simulink model "tracker"  (R2020a)
settings: Solver=VariableStepAuto  StartTime=0.0  StopTime=simulation_time  RelTol=1e-3
values from neighbouring files (symbols this model uses):
  costas_pll_arctan_nstage = 8    [tracker_hw_init.m]
  costas_pll_arctan_point = 16    [tracker_hw_init.m]
  costas_pll_arctan_width = 32    [tracker_hw_init.m]
  DDS_ch_pinc = fc.*(2^(DDS_phase_width)/fs)    [tracker_hw_init.m]
  fs = 120e6    (= 120000000)    [tracker_hw_init.m]
  normalized_EML_power_cordic_nstage = 11    [tracker_hw_init.m]
  normalized_EML_power_cordic_point = 32    [tracker_hw_init.m]
  normalized_EML_power_cordic_width = 32    [tracker_hw_init.m]
  ts = 1/fs    (= 8.33333333333e-09)    [tracker_hw_init.m]
undefined symbols (not defined in the file or in its folder): cacode, i
libraries: xbsIndex_r4 x1873
(part 4 of 14)

== system tracker/CA_code_bank/input_router/address_router32 ==
  ca_select : Inport
  Mux{,1..10} (11 alike) : xbsIndex_r4/Mux  inputs=2  en=off  latency=1  precision=Full  arith_type=Unsigned  n_bits=16  bin_pt=14  quantization=Truncate  overflow=Wrap  dbl_ovrd=off  block_type=mux
  Relational{,1..10} (11 alike) : xbsIndex_r4/Relational  mode=a=b  op_type=Bool  en=off  latency=1  dbl_ovrd=off  block_type=relational
  ca_addr : Outport
  wires:
  [CA_code_addr_ch11] -> Mux10/3
  Mux8/1 -> Mux7/2
  Mux5/1 -> Mux4/2
  [CA_code_select_ch8] -> Relational7/1
  [CA_code_addr_ch9] -> Mux8/3
  [CA_code_select_ch7] -> Relational6/1
  Relational/1 -> Mux/1
  [CA_code_addr_ch1] -> Mux/3
  Mux9/1 -> Mux8/2
  ca_select/1 -> Relational1/2, Relational2/2, Relational3/2, Relational4/2, Relational5/2, Relational6/2, Relational7/2, Relational8/2, Relational9/2, Relational10/2, Relational/2
  Relational9/1 -> Mux9/1
  Mux3/1 -> Mux2/2
  [CA_code_select_ch4] -> Relational3/1
  [CA_code_select_ch3] -> Relational2/1
  Relational8/1 -> Mux8/1
  Relational2/1 -> Mux2/1
  [CA_code_addr_ch5] -> Mux4/3
  [CA_code_select_ch5] -> Relational4/1
  Relational10/1 -> Mux10/1
  Mux2/1 -> Mux1/2
  [CA_code_select_ch2] -> Relational1/1
  Mux4/1 -> Mux3/2
  Relational7/1 -> Mux7/1
  Relational4/1 -> Mux4/1
  [CA_code_select_ch6] -> Relational5/1
  [CA_code_addr_ch6] -> Mux5/3
  [CA_code_addr_ch3] -> Mux2/3
  [CA_code_select_ch1] -> Relational/1
  [CA_code_addr_ch4] -> Mux3/3
  Relational3/1 -> Mux3/1
  [CA_code_select_ch11] -> Relational10/1
  [CA_code_select_ch10] -> Relational9/1
  [CA_code_select_ch9] -> Relational8/1
  Relational5/1 -> Mux5/1
  Mux10/1 -> Mux9/2
  [CA_code_addr_ch10] -> Mux9/3
  Mux7/1 -> Mux6/2
  [CA_code_addr_ch12] -> Mux10/2
  Relational1/1 -> Mux1/1
  [CA_code_addr_ch8] -> Mux7/3
  [CA_code_addr_ch7] -> Mux6/3
  Mux1/1 -> Mux/2
  [CA_code_addr_ch2] -> Mux1/3
  Relational6/1 -> Mux6/1
  Mux6/1 -> Mux5/2
  Mux/1 -> ca_addr/1

== system tracker/CA_code_bank/input_router/address_router33 ==
  ca_select : Inport
  Mux{,1..10} (11 alike) : xbsIndex_r4/Mux  inputs=2  en=off  latency=1  precision=Full  arith_type=Unsigned  n_bits=16  bin_pt=14  quantization=Truncate  overflow=Wrap  dbl_ovrd=off  block_type=mux
  Relational{,1..10} (11 alike) : xbsIndex_r4/Relational  mode=a=b  op_type=Bool  en=off  latency=1  dbl_ovrd=off  block_type=relational
  ca_addr : Outport
  wires:
  Mux/1 -> ca_addr/1
  Mux6/1 -> Mux5/2
  Relational6/1 -> Mux6/1
  [CA_code_addr_ch2] -> Mux1/3
  Mux1/1 -> Mux/2
  [CA_code_addr_ch7] -> Mux6/3
  [CA_code_addr_ch8] -> Mux7/3
  Relational1/1 -> Mux1/1
  [CA_code_addr_ch12] -> Mux10/2
  Mux7/1 -> Mux6/2
  [CA_code_addr_ch10] -> Mux9/3
  Mux10/1 -> Mux9/2
  Relational5/1 -> Mux5/1
  [CA_code_select_ch9] -> Relational8/1
  [CA_code_select_ch10] -> Relational9/1
  [CA_code_select_ch11] -> Relational10/1
  Relational3/1 -> Mux3/1
  [CA_code_addr_ch4] -> Mux3/3
  [CA_code_select_ch1] -> Relational/1
  [CA_code_addr_ch3] -> Mux2/3
  [CA_code_addr_ch6] -> Mux5/3
  [CA_code_select_ch6] -> Relational5/1
  Relational4/1 -> Mux4/1
  Relational7/1 -> Mux7/1
  Mux4/1 -> Mux3/2
  [CA_code_select_ch2] -> Relational1/1
  Mux2/1 -> Mux1/2
  Relational10/1 -> Mux10/1
  [CA_code_select_ch5] -> Relational4/1
  [CA_code_addr_ch5] -> Mux4/3
  Relational2/1 -> Mux2/1
  Relational8/1 -> Mux8/1
  [CA_code_select_ch3] -> Relational2/1
  [CA_code_select_ch4] -> Relational3/1
  Mux3/1 -> Mux2/2
  Relational9/1 -> Mux9/1
  ca_select/1 -> Relational/2, Relational10/2, Relational9/2, Relational8/2, Relational7/2, Relational6/2, Relational5/2, Relational4/2, Relational3/2, Relational2/2, Relational1/2
  Mux9/1 -> Mux8/2
  [CA_code_addr_ch1] -> Mux/3
  Relational/1 -> Mux/1
  [CA_code_select_ch7] -> Relational6/1
  [CA_code_addr_ch9] -> Mux8/3
  [CA_code_select_ch8] -> Relational7/1
  Mux5/1 -> Mux4/2
  Mux8/1 -> Mux7/2
  [CA_code_addr_ch11] -> Mux10/3

== system tracker/CA_code_bank/input_router/address_router34 ==
  ca_select : Inport
  Mux{,1..10} (11 alike) : xbsIndex_r4/Mux  inputs=2  en=off  latency=1  precision=Full  arith_type=Unsigned  n_bits=16  bin_pt=14  quantization=Truncate  overflow=Wrap  dbl_ovrd=off  block_type=mux
  Relational{,1..10} (11 alike) : xbsIndex_r4/Relational  mode=a=b  op_type=Bool  en=off  latency=1  dbl_ovrd=off  block_type=relational
  ca_addr : Outport
  wires:
  Mux/1 -> ca_addr/1
  Mux6/1 -> Mux5/2
  Relational6/1 -> Mux6/1
  [CA_code_addr_ch2] -> Mux1/3
  Mux1/1 -> Mux/2
  [CA_code_addr_ch7] -> Mux6/3
  [CA_code_addr_ch8] -> Mux7/3
  Relational1/1 -> Mux1/1
  [CA_code_addr_ch12] -> Mux10/2
  Mux7/1 -> Mux6/2
  [CA_code_addr_ch10] -> Mux9/3
  Mux10/1 -> Mux9/2
  Relational5/1 -> Mux5/1
  [CA_code_select_ch9] -> Relational8/1
  [CA_code_select_ch10] -> Relational9/1
  [CA_code_select_ch11] -> Relational10/1
  Relational3/1 -> Mux3/1
  [CA_code_addr_ch4] -> Mux3/3
  [CA_code_select_ch1] -> Relational/1
  [CA_code_addr_ch3] -> Mux2/3
  [CA_code_addr_ch6] -> Mux5/3
  [CA_code_select_ch6] -> Relational5/1
  Relational4/1 -> Mux4/1
  Relational7/1 -> Mux7/1
  Mux4/1 -> Mux3/2
  [CA_code_select_ch2] -> Relational1/1
  Mux2/1 -> Mux1/2
  Relational10/1 -> Mux10/1
  [CA_code_select_ch5] -> Relational4/1
  [CA_code_addr_ch5] -> Mux4/3
  Relational2/1 -> Mux2/1
  Relational8/1 -> Mux8/1
  [CA_code_select_ch3] -> Relational2/1
  [CA_code_select_ch4] -> Relational3/1
  Mux3/1 -> Mux2/2
  Relational9/1 -> Mux9/1
  ca_select/1 -> Relational/2, Relational10/2, Relational9/2, Relational8/2, Relational7/2, Relational6/2, Relational5/2, Relational4/2, Relational3/2, Relational2/2, Relational1/2
  Mux9/1 -> Mux8/2
  [CA_code_addr_ch1] -> Mux/3
  Relational/1 -> Mux/1
  [CA_code_select_ch7] -> Relational6/1
  [CA_code_addr_ch9] -> Mux8/3
  [CA_code_select_ch8] -> Relational7/1
  Mux5/1 -> Mux4/2
  Mux8/1 -> Mux7/2
  [CA_code_addr_ch11] -> Mux10/3

== system tracker/CA_code_bank/input_router/address_router35 ==
  ca_select : Inport
  Mux{,1..10} (11 alike) : xbsIndex_r4/Mux  inputs=2  en=off  latency=1  precision=Full  arith_type=Unsigned  n_bits=16  bin_pt=14  quantization=Truncate  overflow=Wrap  dbl_ovrd=off  block_type=mux
  Relational{,1..10} (11 alike) : xbsIndex_r4/Relational  mode=a=b  op_type=Bool  en=off  latency=1  dbl_ovrd=off  block_type=relational
  ca_addr : Outport
  wires:
  [CA_code_addr_ch11] -> Mux10/3
  Mux8/1 -> Mux7/2
  Mux5/1 -> Mux4/2
  [CA_code_select_ch8] -> Relational7/1
  [CA_code_addr_ch9] -> Mux8/3
  [CA_code_select_ch7] -> Relational6/1
  Relational/1 -> Mux/1
  [CA_code_addr_ch1] -> Mux/3
  Mux9/1 -> Mux8/2
  ca_select/1 -> Relational1/2, Relational2/2, Relational3/2, Relational4/2, Relational5/2, Relational6/2, Relational7/2, Relational8/2, Relational9/2, Relational10/2, Relational/2
  Relational9/1 -> Mux9/1
  Mux3/1 -> Mux2/2
  [CA_code_select_ch4] -> Relational3/1
  [CA_code_select_ch3] -> Relational2/1
  Relational8/1 -> Mux8/1
  Relational2/1 -> Mux2/1
  [CA_code_addr_ch5] -> Mux4/3
  [CA_code_select_ch5] -> Relational4/1
  Relational10/1 -> Mux10/1
  Mux2/1 -> Mux1/2
  [CA_code_select_ch2] -> Relational1/1
  Mux4/1 -> Mux3/2
  Relational7/1 -> Mux7/1
  Relational4/1 -> Mux4/1
  [CA_code_select_ch6] -> Relational5/1
  [CA_code_addr_ch6] -> Mux5/3
  [CA_code_addr_ch3] -> Mux2/3
  [CA_code_select_ch1] -> Relational/1
  [CA_code_addr_ch4] -> Mux3/3
  Relational3/1 -> Mux3/1
  [CA_code_select_ch11] -> Relational10/1
  [CA_code_select_ch10] -> Relational9/1
  [CA_code_select_ch9] -> Relational8/1
  Relational5/1 -> Mux5/1
  Mux10/1 -> Mux9/2
  [CA_code_addr_ch10] -> Mux9/3
  Mux7/1 -> Mux6/2
  [CA_code_addr_ch12] -> Mux10/2
  Relational1/1 -> Mux1/1
  [CA_code_addr_ch8] -> Mux7/3
  [CA_code_addr_ch7] -> Mux6/3
  Mux1/1 -> Mux/2
  [CA_code_addr_ch2] -> Mux1/3
  Relational6/1 -> Mux6/1
  Mux6/1 -> Mux5/2
  Mux/1 -> ca_addr/1

== system tracker/CA_code_bank/input_router/address_router36 ==
  ca_select : Inport
  Mux{,1..10} (11 alike) : xbsIndex_r4/Mux  inputs=2  en=off  latency=1  precision=Full  arith_type=Unsigned  n_bits=16  bin_pt=14  quantization=Truncate  overflow=Wrap  dbl_ovrd=off  block_type=mux
  Relational{,1..10} (11 alike) : xbsIndex_r4/Relational  mode=a=b  op_type=Bool  en=off  latency=1  dbl_ovrd=off  block_type=relational
  ca_addr : Outport
  wires:
  Mux/1 -> ca_addr/1
  Mux6/1 -> Mux5/2
  Relational6/1 -> Mux6/1
  [CA_code_addr_ch2] -> Mux1/3
  Mux1/1 -> Mux/2
  [CA_code_addr_ch7] -> Mux6/3
  [CA_code_addr_ch8] -> Mux7/3
  Relational1/1 -> Mux1/1
  [CA_code_addr_ch12] -> Mux10/2
  Mux7/1 -> Mux6/2
  [CA_code_addr_ch10] -> Mux9/3
  Mux10/1 -> Mux9/2
  Relational5/1 -> Mux5/1
  [CA_code_select_ch9] -> Relational8/1
  [CA_code_select_ch10] -> Relational9/1
  [CA_code_select_ch11] -> Relational10/1
  Relational3/1 -> Mux3/1
  [CA_code_addr_ch4] -> Mux3/3
  [CA_code_select_ch1] -> Relational/1
  [CA_code_addr_ch3] -> Mux2/3
  [CA_code_addr_ch6] -> Mux5/3
  [CA_code_select_ch6] -> Relational5/1
  Relational4/1 -> Mux4/1
  Relational7/1 -> Mux7/1
  Mux4/1 -> Mux3/2
  [CA_code_select_ch2] -> Relational1/1
  Mux2/1 -> Mux1/2
  Relational10/1 -> Mux10/1
  [CA_code_select_ch5] -> Relational4/1
  [CA_code_addr_ch5] -> Mux4/3
  Relational2/1 -> Mux2/1
  Relational8/1 -> Mux8/1
  [CA_code_select_ch3] -> Relational2/1
  [CA_code_select_ch4] -> Relational3/1
  Mux3/1 -> Mux2/2
  Relational9/1 -> Mux9/1
  ca_select/1 -> Relational/2, Relational10/2, Relational9/2, Relational8/2, Relational7/2, Relational6/2, Relational5/2, Relational4/2, Relational3/2, Relational2/2, Relational1/2
  Mux9/1 -> Mux8/2
  [CA_code_addr_ch1] -> Mux/3
  Relational/1 -> Mux/1
  [CA_code_select_ch7] -> Relational6/1
  [CA_code_addr_ch9] -> Mux8/3
  [CA_code_select_ch8] -> Relational7/1
  Mux5/1 -> Mux4/2
  Mux8/1 -> Mux7/2
  [CA_code_addr_ch11] -> Mux10/3

== system tracker/CA_code_bank/input_router/address_router37 ==
  ca_select : Inport
  Mux{,1..10} (11 alike) : xbsIndex_r4/Mux  inputs=2  en=off  latency=1  precision=Full  arith_type=Unsigned  n_bits=16  bin_pt=14  quantization=Truncate  overflow=Wrap  dbl_ovrd=off  block_type=mux
  Relational{,1..10} (11 alike) : xbsIndex_r4/Relational  mode=a=b  op_type=Bool  en=off  latency=1  dbl_ovrd=off  block_type=relational
  ca_addr : Outport
  wires:
  Mux/1 -> ca_addr/1
  Mux6/1 -> Mux5/2
  Relational6/1 -> Mux6/1
  [CA_code_addr_ch2] -> Mux1/3
  Mux1/1 -> Mux/2
  [CA_code_addr_ch7] -> Mux6/3
  [CA_code_addr_ch8] -> Mux7/3
  Relational1/1 -> Mux1/1
  [CA_code_addr_ch12] -> Mux10/2
  Mux7/1 -> Mux6/2
  [CA_code_addr_ch10] -> Mux9/3
  Mux10/1 -> Mux9/2
  Relational5/1 -> Mux5/1
  [CA_code_select_ch9] -> Relational8/1
  [CA_code_select_ch10] -> Relational9/1
  [CA_code_select_ch11] -> Relational10/1
  Relational3/1 -> Mux3/1
  [CA_code_addr_ch4] -> Mux3/3
  [CA_code_select_ch1] -> Relational/1
  [CA_code_addr_ch3] -> Mux2/3
  [CA_code_addr_ch6] -> Mux5/3
  [CA_code_select_ch6] -> Relational5/1
  Relational4/1 -> Mux4/1
  Relational7/1 -> Mux7/1
  Mux4/1 -> Mux3/2
  [CA_code_select_ch2] -> Relational1/1
  Mux2/1 -> Mux1/2
  Relational10/1 -> Mux10/1
  [CA_code_select_ch5] -> Relational4/1
  [CA_code_addr_ch5] -> Mux4/3
  Relational2/1 -> Mux2/1
  Relational8/1 -> Mux8/1
  [CA_code_select_ch3] -> Relational2/1
  [CA_code_select_ch4] -> Relational3/1
  Mux3/1 -> Mux2/2
  Relational9/1 -> Mux9/1
  ca_select/1 -> Relational/2, Relational10/2, Relational9/2, Relational8/2, Relational7/2, Relational6/2, Relational5/2, Relational4/2, Relational3/2, Relational2/2, Relational1/2
  Mux9/1 -> Mux8/2
  [CA_code_addr_ch1] -> Mux/3
  Relational/1 -> Mux/1
  [CA_code_select_ch7] -> Relational6/1
  [CA_code_addr_ch9] -> Mux8/3
  [CA_code_select_ch8] -> Relational7/1
  Mux5/1 -> Mux4/2
  Mux8/1 -> Mux7/2
  [CA_code_addr_ch11] -> Mux10/3

== system tracker/CA_code_bank/input_router/address_router4 ==
  ca_select : Inport
  Mux{,1..10} (11 alike) : xbsIndex_r4/Mux  inputs=2  en=off  latency=1  precision=Full  arith_type=Unsigned  n_bits=16  bin_pt=14  quantization=Truncate  overflow=Wrap  dbl_ovrd=off  block_type=mux
  Relational{,1..10} (11 alike) : xbsIndex_r4/Relational  mode=a=b  op_type=Bool  en=off  latency=1  dbl_ovrd=off  block_type=relational
  ca_addr : Outport
  wires:
  Mux/1 -> ca_addr/1
  Mux6/1 -> Mux5/2
  Relational6/1 -> Mux6/1
  [CA_code_addr_ch2] -> Mux1/3
  Mux1/1 -> Mux/2
  [CA_code_addr_ch7] -> Mux6/3
  [CA_code_addr_ch8] -> Mux7/3
  Relational1/1 -> Mux1/1
  [CA_code_addr_ch12] -> Mux10/2
  Mux7/1 -> Mux6/2
  [CA_code_addr_ch10] -> Mux9/3
  Mux10/1 -> Mux9/2
  Relational5/1 -> Mux5/1
  [CA_code_select_ch9] -> Relational8/1
  [CA_code_select_ch10] -> Relational9/1
  [CA_code_select_ch11] -> Relational10/1
  Relational3/1 -> Mux3/1
  [CA_code_addr_ch4] -> Mux3/3
  [CA_code_select_ch1] -> Relational/1
  [CA_code_addr_ch3] -> Mux2/3
  [CA_code_addr_ch6] -> Mux5/3
  [CA_code_select_ch6] -> Relational5/1
  Relational4/1 -> Mux4/1
  Relational7/1 -> Mux7/1
  Mux4/1 -> Mux3/2
  [CA_code_select_ch2] -> Relational1/1
  Mux2/1 -> Mux1/2
  Relational10/1 -> Mux10/1
  [CA_code_select_ch5] -> Relational4/1
  [CA_code_addr_ch5] -> Mux4/3
  Relational2/1 -> Mux2/1
  Relational8/1 -> Mux8/1
  [CA_code_select_ch3] -> Relational2/1
  [CA_code_select_ch4] -> Relational3/1
  Mux3/1 -> Mux2/2
  Relational9/1 -> Mux9/1
  ca_select/1 -> Relational/2, Relational10/2, Relational9/2, Relational8/2, Relational7/2, Relational6/2, Relational5/2, Relational4/2, Relational3/2, Relational2/2, Relational1/2
  Mux9/1 -> Mux8/2
  [CA_code_addr_ch1] -> Mux/3
  Relational/1 -> Mux/1
  [CA_code_select_ch7] -> Relational6/1
  [CA_code_addr_ch9] -> Mux8/3
  [CA_code_select_ch8] -> Relational7/1
  Mux5/1 -> Mux4/2
  Mux8/1 -> Mux7/2
  [CA_code_addr_ch11] -> Mux10/3

== system tracker/CA_code_bank/input_router/address_router5 ==
  ca_select : Inport
  Mux{,1..10} (11 alike) : xbsIndex_r4/Mux  inputs=2  en=off  latency=1  precision=Full  arith_type=Unsigned  n_bits=16  bin_pt=14  quantization=Truncate  overflow=Wrap  dbl_ovrd=off  block_type=mux
  Relational{,1..10} (11 alike) : xbsIndex_r4/Relational  mode=a=b  op_type=Bool  en=off  latency=1  dbl_ovrd=off  block_type=relational
  ca_addr : Outport
  wires:
  [CA_code_addr_ch11] -> Mux10/3
  Mux8/1 -> Mux7/2
  Mux5/1 -> Mux4/2
  [CA_code_select_ch8] -> Relational7/1
  [CA_code_addr_ch9] -> Mux8/3
  [CA_code_select_ch7] -> Relational6/1
  Relational/1 -> Mux/1
  [CA_code_addr_ch1] -> Mux/3
  Mux9/1 -> Mux8/2
  ca_select/1 -> Relational1/2, Relational2/2, Relational3/2, Relational4/2, Relational5/2, Relational6/2, Relational7/2, Relational8/2, Relational9/2, Relational10/2, Relational/2
  Relational9/1 -> Mux9/1
  Mux3/1 -> Mux2/2
  [CA_code_select_ch4] -> Relational3/1
  [CA_code_select_ch3] -> Relational2/1
  Relational8/1 -> Mux8/1
  Relational2/1 -> Mux2/1
  [CA_code_addr_ch5] -> Mux4/3
  [CA_code_select_ch5] -> Relational4/1
  Relational10/1 -> Mux10/1
  Mux2/1 -> Mux1/2
  [CA_code_select_ch2] -> Relational1/1
  Mux4/1 -> Mux3/2
  Relational7/1 -> Mux7/1
  Relational4/1 -> Mux4/1
  [CA_code_select_ch6] -> Relational5/1
  [CA_code_addr_ch6] -> Mux5/3
  [CA_code_addr_ch3] -> Mux2/3
  [CA_code_select_ch1] -> Relational/1
  [CA_code_addr_ch4] -> Mux3/3
  Relational3/1 -> Mux3/1
  [CA_code_select_ch11] -> Relational10/1
  [CA_code_select_ch10] -> Relational9/1
  [CA_code_select_ch9] -> Relational8/1
  Relational5/1 -> Mux5/1
  Mux10/1 -> Mux9/2
  [CA_code_addr_ch10] -> Mux9/3
  Mux7/1 -> Mux6/2
  [CA_code_addr_ch12] -> Mux10/2
  Relational1/1 -> Mux1/1
  [CA_code_addr_ch8] -> Mux7/3
  [CA_code_addr_ch7] -> Mux6/3
  Mux1/1 -> Mux/2
  [CA_code_addr_ch2] -> Mux1/3
  Relational6/1 -> Mux6/1
  Mux6/1 -> Mux5/2
  Mux/1 -> ca_addr/1

== system tracker/CA_code_bank/input_router/address_router6 ==
  ca_select : Inport
  Mux{,1..10} (11 alike) : xbsIndex_r4/Mux  inputs=2  en=off  latency=1  precision=Full  arith_type=Unsigned  n_bits=16  bin_pt=14  quantization=Truncate  overflow=Wrap  dbl_ovrd=off  block_type=mux
  Relational{,1..10} (11 alike) : xbsIndex_r4/Relational  mode=a=b  op_type=Bool  en=off  latency=1  dbl_ovrd=off  block_type=relational
  ca_addr : Outport
  wires:
  Mux/1 -> ca_addr/1
  Mux6/1 -> Mux5/2
  Relational6/1 -> Mux6/1
  [CA_code_addr_ch2] -> Mux1/3
  Mux1/1 -> Mux/2
  [CA_code_addr_ch7] -> Mux6/3
  [CA_code_addr_ch8] -> Mux7/3
  Relational1/1 -> Mux1/1
  [CA_code_addr_ch12] -> Mux10/2
  Mux7/1 -> Mux6/2
  [CA_code_addr_ch10] -> Mux9/3
  Mux10/1 -> Mux9/2
  Relational5/1 -> Mux5/1
  [CA_code_select_ch9] -> Relational8/1
  [CA_code_select_ch10] -> Relational9/1
  [CA_code_select_ch11] -> Relational10/1
  Relational3/1 -> Mux3/1
  [CA_code_addr_ch4] -> Mux3/3
  [CA_code_select_ch1] -> Relational/1
  [CA_code_addr_ch3] -> Mux2/3
  [CA_code_addr_ch6] -> Mux5/3
  [CA_code_select_ch6] -> Relational5/1
  Relational4/1 -> Mux4/1
  Relational7/1 -> Mux7/1
  Mux4/1 -> Mux3/2
  [CA_code_select_ch2] -> Relational1/1
  Mux2/1 -> Mux1/2
  Relational10/1 -> Mux10/1
  [CA_code_select_ch5] -> Relational4/1
  [CA_code_addr_ch5] -> Mux4/3
  Relational2/1 -> Mux2/1
  Relational8/1 -> Mux8/1
  [CA_code_select_ch3] -> Relational2/1
  [CA_code_select_ch4] -> Relational3/1
  Mux3/1 -> Mux2/2
  Relational9/1 -> Mux9/1
  ca_select/1 -> Relational/2, Relational10/2, Relational9/2, Relational8/2, Relational7/2, Relational6/2, Relational5/2, Relational4/2, Relational3/2, Relational2/2, Relational1/2
  Mux9/1 -> Mux8/2
  [CA_code_addr_ch1] -> Mux/3
  Relational/1 -> Mux/1
  [CA_code_select_ch7] -> Relational6/1
  [CA_code_addr_ch9] -> Mux8/3
  [CA_code_select_ch8] -> Relational7/1
  Mux5/1 -> Mux4/2
  Mux8/1 -> Mux7/2
  [CA_code_addr_ch11] -> Mux10/3

== system tracker/CA_code_bank/input_router/address_router7 ==
  ca_select : Inport
  Mux{,1..10} (11 alike) : xbsIndex_r4/Mux  inputs=2  en=off  latency=1  precision=Full  arith_type=Unsigned  n_bits=16  bin_pt=14  quantization=Truncate  overflow=Wrap  dbl_ovrd=off  block_type=mux
  Relational{,1..10} (11 alike) : xbsIndex_r4/Relational  mode=a=b  op_type=Bool  en=off  latency=1  dbl_ovrd=off  block_type=relational
  ca_addr : Outport
  wires:
  Mux/1 -> ca_addr/1
  Mux6/1 -> Mux5/2
  Relational6/1 -> Mux6/1
  [CA_code_addr_ch2] -> Mux1/3
  Mux1/1 -> Mux/2
  [CA_code_addr_ch7] -> Mux6/3
  [CA_code_addr_ch8] -> Mux7/3
  Relational1/1 -> Mux1/1
  [CA_code_addr_ch12] -> Mux10/2
  Mux7/1 -> Mux6/2
  [CA_code_addr_ch10] -> Mux9/3
  Mux10/1 -> Mux9/2
  Relational5/1 -> Mux5/1
  [CA_code_select_ch9] -> Relational8/1
  [CA_code_select_ch10] -> Relational9/1
  [CA_code_select_ch11] -> Relational10/1
  Relational3/1 -> Mux3/1
  [CA_code_addr_ch4] -> Mux3/3
  [CA_code_select_ch1] -> Relational/1
  [CA_code_addr_ch3] -> Mux2/3
  [CA_code_addr_ch6] -> Mux5/3
  [CA_code_select_ch6] -> Relational5/1
  Relational4/1 -> Mux4/1
  Relational7/1 -> Mux7/1
  Mux4/1 -> Mux3/2
  [CA_code_select_ch2] -> Relational1/1
  Mux2/1 -> Mux1/2
  Relational10/1 -> Mux10/1
  [CA_code_select_ch5] -> Relational4/1
  [CA_code_addr_ch5] -> Mux4/3
  Relational2/1 -> Mux2/1
  Relational8/1 -> Mux8/1
  [CA_code_select_ch3] -> Relational2/1
  [CA_code_select_ch4] -> Relational3/1
  Mux3/1 -> Mux2/2
  Relational9/1 -> Mux9/1
  ca_select/1 -> Relational/2, Relational10/2, Relational9/2, Relational8/2, Relational7/2, Relational6/2, Relational5/2, Relational4/2, Relational3/2, Relational2/2, Relational1/2
  Mux9/1 -> Mux8/2
  [CA_code_addr_ch1] -> Mux/3
  Relational/1 -> Mux/1
  [CA_code_select_ch7] -> Relational6/1
  [CA_code_addr_ch9] -> Mux8/3
  [CA_code_select_ch8] -> Relational7/1
  Mux5/1 -> Mux4/2
  Mux8/1 -> Mux7/2
  [CA_code_addr_ch11] -> Mux10/3

== system tracker/CA_code_bank/input_router/address_router8 ==
  ca_select : Inport
  Mux{,1..10} (11 alike) : xbsIndex_r4/Mux  inputs=2  en=off  latency=1  precision=Full  arith_type=Unsigned  n_bits=16  bin_pt=14  quantization=Truncate  overflow=Wrap  dbl_ovrd=off  block_type=mux
  Relational{,1..10} (11 alike) : xbsIndex_r4/Relational  mode=a=b  op_type=Bool  en=off  latency=1  dbl_ovrd=off  block_type=relational
  ca_addr : Outport
  wires:
  [CA_code_addr_ch11] -> Mux10/3
  Mux8/1 -> Mux7/2
  Mux5/1 -> Mux4/2
  [CA_code_select_ch8] -> Relational7/1
  [CA_code_addr_ch9] -> Mux8/3
  [CA_code_select_ch7] -> Relational6/1
  Relational/1 -> Mux/1
  [CA_code_addr_ch1] -> Mux/3
  Mux9/1 -> Mux8/2
  ca_select/1 -> Relational1/2, Relational2/2, Relational3/2, Relational4/2, Relational5/2, Relational6/2, Relational7/2, Relational8/2, Relational9/2, Relational10/2, Relational/2
  Relational9/1 -> Mux9/1
  Mux3/1 -> Mux2/2
  [CA_code_select_ch4] -> Relational3/1
  [CA_code_select_ch3] -> Relational2/1
  Relational8/1 -> Mux8/1
  Relational2/1 -> Mux2/1
  [CA_code_addr_ch5] -> Mux4/3
  [CA_code_select_ch5] -> Relational4/1
  Relational10/1 -> Mux10/1
  Mux2/1 -> Mux1/2
  [CA_code_select_ch2] -> Relational1/1
  Mux4/1 -> Mux3/2
  Relational7/1 -> Mux7/1
  Relational4/1 -> Mux4/1
  [CA_code_select_ch6] -> Relational5/1
  [CA_code_addr_ch6] -> Mux5/3
  [CA_code_addr_ch3] -> Mux2/3
  [CA_code_select_ch1] -> Relational/1
  [CA_code_addr_ch4] -> Mux3/3
  Relational3/1 -> Mux3/1
  [CA_code_select_ch11] -> Relational10/1
  [CA_code_select_ch10] -> Relational9/1
  [CA_code_select_ch9] -> Relational8/1
  Relational5/1 -> Mux5/1
  Mux10/1 -> Mux9/2
  [CA_code_addr_ch10] -> Mux9/3
  Mux7/1 -> Mux6/2
  [CA_code_addr_ch12] -> Mux10/2
  Relational1/1 -> Mux1/1
  [CA_code_addr_ch8] -> Mux7/3
  [CA_code_addr_ch7] -> Mux6/3
  Mux1/1 -> Mux/2
  [CA_code_addr_ch2] -> Mux1/3
  Relational6/1 -> Mux6/1
  Mux6/1 -> Mux5/2
  Mux/1 -> ca_addr/1

== system tracker/CA_code_bank/input_router/address_router9 ==
  ca_select : Inport
  Mux{,1..10} (11 alike) : xbsIndex_r4/Mux  inputs=2  en=off  latency=1  precision=Full  arith_type=Unsigned  n_bits=16  bin_pt=14  quantization=Truncate  overflow=Wrap  dbl_ovrd=off  block_type=mux
  Relational{,1..10} (11 alike) : xbsIndex_r4/Relational  mode=a=b  op_type=Bool  en=off  latency=1  dbl_ovrd=off  block_type=relational
  ca_addr : Outport
  wires:
  Mux/1 -> ca_addr/1
  Mux6/1 -> Mux5/2
  Relational6/1 -> Mux6/1
  [CA_code_addr_ch2] -> Mux1/3
  Mux1/1 -> Mux/2
  [CA_code_addr_ch7] -> Mux6/3
  [CA_code_addr_ch8] -> Mux7/3
  Relational1/1 -> Mux1/1
  [CA_code_addr_ch12] -> Mux10/2
  Mux7/1 -> Mux6/2
  [CA_code_addr_ch10] -> Mux9/3
  Mux10/1 -> Mux9/2
  Relational5/1 -> Mux5/1
  [CA_code_select_ch9] -> Relational8/1
  [CA_code_select_ch10] -> Relational9/1
  [CA_code_select_ch11] -> Relational10/1
  Relational3/1 -> Mux3/1
  [CA_code_addr_ch4] -> Mux3/3
  [CA_code_select_ch1] -> Relational/1
  [CA_code_addr_ch3] -> Mux2/3
  [CA_code_addr_ch6] -> Mux5/3
  [CA_code_select_ch6] -> Relational5/1
  Relational4/1 -> Mux4/1
  Relational7/1 -> Mux7/1
  Mux4/1 -> Mux3/2
  [CA_code_select_ch2] -> Relational1/1
  Mux2/1 -> Mux1/2
  Relational10/1 -> Mux10/1
  [CA_code_select_ch5] -> Relational4/1
  [CA_code_addr_ch5] -> Mux4/3
  Relational2/1 -> Mux2/1
  Relational8/1 -> Mux8/1
  [CA_code_select_ch3] -> Relational2/1
  [CA_code_select_ch4] -> Relational3/1
  Mux3/1 -> Mux2/2
  Relational9/1 -> Mux9/1
  ca_select/1 -> Relational/2, Relational10/2, Relational9/2, Relational8/2, Relational7/2, Relational6/2, Relational5/2, Relational4/2, Relational3/2, Relational2/2, Relational1/2
  Mux9/1 -> Mux8/2
  [CA_code_addr_ch1] -> Mux/3
  Relational/1 -> Mux/1
  [CA_code_select_ch7] -> Relational6/1
  [CA_code_addr_ch9] -> Mux8/3
  [CA_code_select_ch8] -> Relational7/1
  Mux5/1 -> Mux4/2
  Mux8/1 -> Mux7/2
  [CA_code_addr_ch11] -> Mux10/3

== system tracker/code_carrier_tracking_loop1/carrier_loop_discriminator/loop_filter ==
  phi : Inport
  AddSub : xbsIndex_r4/AddSub  mode=Addition  use_carryin=off  use_carryout=off  en=off  latency=1  precision=Full  arith_type=Unsigned  n_bits=16  bin_pt=14  quantization=Truncate  overflow=Wrap  use_behavioral_HDL=off  hw_selection=Fabric  pipelined=off  dbl_ovrd=off  block_type=addsub
  AddSub1 : xbsIndex_r4/AddSub  mode=Addition  use_carryin=off  use_carryout=off  en=off  latency=1  precision=Full  arith_type=Unsigned  n_bits=16  bin_pt=14  quantization=Truncate  overflow=Wrap  use_behavioral_HDL=off  hw_selection=Fabric  pipelined=off  dbl_ovrd=off  block_type=addsub
  Mux : xbsIndex_r4/Mux  inputs=2  en=off  latency=1  precision=Full  arith_type=Unsigned  n_bits=16  bin_pt=14  quantization=Truncate  overflow=Wrap  dbl_ovrd=off  block_type=mux
  Mux2 : xbsIndex_r4/Mux  inputs=2  en=off  latency=1  precision=Full  arith_type=Unsigned  n_bits=16  bin_pt=14  quantization=Truncate  overflow=Wrap  dbl_ovrd=off  block_type=mux
  a3w0 : xbsIndex_r4/CMult  const=1  gui_display_data_type=Fixed-point  const_n_bits=16  const_bin_pt=14  float_type=Single  exp_bits=8  fraction_bits=24  en=off  latency=1  precision=Full  arith_type="Signed  (2's comp)"  n_bits=16  bin_pt=14  quantization=Truncate  overflow=Wrap  use_behavioral_HDL=off  mem_type=Distributed RAM  pipeline=off  dbl_ovrd=off  block_type=cmult
  a3w2 : xbsIndex_r4/CMult  const=1  gui_display_data_type=Fixed-point  const_n_bits=16  const_bin_pt=14  float_type=Single  exp_bits=8  fraction_bits=24  en=off  latency=1  precision=Full  arith_type="Signed  (2's comp)"  n_bits=16  bin_pt=14  quantization=Truncate  overflow=Wrap  use_behavioral_HDL=off  mem_type=Distributed RAM  pipeline=off  dbl_ovrd=off  block_type=cmult
  digital_bilinear_z_transform_integrator : Subsystem
  digital_bilinear_z_transform_integrator1 : Subsystem
  digital_bilinear_z_transform_integrator2 : Subsystem
  w3 : xbsIndex_r4/CMult  const=1  gui_display_data_type=Fixed-point  const_n_bits=16  const_bin_pt=14  float_type=Single  exp_bits=8  fraction_bits=24  en=off  latency=1  precision=Full  arith_type="Signed  (2's comp)"  n_bits=16  bin_pt=14  quantization=Truncate  overflow=Wrap  use_behavioral_HDL=off  mem_type=Distributed RAM  pipeline=off  dbl_ovrd=off  block_type=cmult
  to_nco : Outport
  wires:
  phi/1 -> a3w0/1, a3w2/1, w3/1
  w3/1 -> digital_bilinear_z_transform_integrator2/1(x[n])
  digital_bilinear_z_transform_integrator2/1(y[n]) -> Mux/2, AddSub/1
  AddSub/1 -> Mux/3
  a3w2/1 -> AddSub/2
  Mux/1 -> digital_bilinear_z_transform_integrator/1(x[n])
  Mux2/1 -> digital_bilinear_z_transform_integrator1/1(x[n])
  a3w0/1 -> AddSub1/2
  AddSub1/1 -> Mux2/3
  digital_bilinear_z_transform_integrator/1(y[n]) -> AddSub1/1, Mux2/2
  digital_bilinear_z_transform_integrator1/1(y[n]) -> to_nco/1

== system tracker/code_carrier_tracking_loop1/carrier_loop_discriminator/pll_discriminators ==
  I : Inport
  Q : Inport  Port=2
  Mux : xbsIndex_r4/Mux  inputs=3  en=off  latency=1  precision=Full  arith_type=Unsigned  n_bits=16  bin_pt=14  quantization=Truncate  overflow=Wrap  dbl_ovrd=off  block_type=mux
  costas_pll_QI : Subsystem
  costas_pll_arctan : Subsystem
  costas_pll_sign : Subsystem
  phi : Outport
  wires:
  costas_pll_QI/1(sin(2*phi)) -> Mux/4
  I/1 -> costas_pll_arctan/1(I), costas_pll_QI/1(I), costas_pll_sign/1(I)
  Q/1 -> costas_pll_arctan/2(Q), costas_pll_QI/2(Q), costas_pll_sign/2(Q)
  costas_pll_sign/1(sin(phi)) -> Mux/3
  costas_pll_arctan/1(phi) -> Mux/2
  Mux/1 -> phi/1

== system tracker/code_carrier_tracking_loop1/code_loop_discriminator/DLL_Discriminators ==
  Ies : Inport
  Qes : Inport  Port=2
  Ils : Inport  Port=3
  Qls : Inport  Port=4
  EML_power : Subsystem
  Ies1 : InportShadow
  Ils1 : InportShadow  Port=3
  Mult{,1..3} (4 alike) : xbsIndex_r4/Mult  precision=User Defined  arith_type="Signed  (2's comp)"  n_bits=DLL_Discriminators_mult_width  bin_pt=DLL_Discriminators_mult_point  quantization="Round  (unbiased: +/- Inf)"  overflow=Saturate  en=off  latency=3  use_behavioral_HDL=off  opt=Speed  use_embedded=on  optimum_pipeline=off  pipeline=on  dbl_ovrd=off  use_rpm=on  placement_style=Triangular  block_type=mult
  Mux : xbsIndex_r4/Mux  inputs=3  en=off  latency=1  precision=Full  arith_type=Unsigned  n_bits=16  bin_pt=14  quantization=Truncate  overflow=Wrap  dbl_ovrd=off  block_type=mux
  coherent_discriminator : xbsIndex_r4/AddSub  mode=Subtraction  use_carryin=off  use_carryout=off  en=off  latency=1  precision=User Defined  arith_type="Signed  (2's comp)"  n_bits=coherent_discriminator_width  bin_pt=coherent_discriminator_point  quantization="Round  (unbiased: +/- Inf)"  overflow=Saturate  use_behavioral_HDL=off  hw_selection=Fabric  pipelined=off  dbl_ovrd=off  block_type=addsub
  normalized_EML_power : Subsystem
  sdfa : Outport
  wires:
  Ils/1 -> Mult2/2, Mult2/1
  Ies/1 -> Mult/1, Mult/2
  Qes/1 -> Mult1/2, Mult1/1
  Qls/1 -> Mult3/2, Mult3/1
  Mult/1 -> [Ies2]
  Mult2/1 -> [Ils2]
  Mult1/1 -> [Qes2]
  Mult3/1 -> [Qls2]
  Ils1/1 -> coherent_discriminator/2
  Ies1/1 -> coherent_discriminator/1
  [Qls2] -> EML_power/4(Qls2)
  [Ils2] -> EML_power/3(Ils2)
  [Qes2] -> EML_power/2(Qes2)
  [Ies2] -> EML_power/1(Ies2)
  [Ies2] -> normalized_EML_power/1(Ies2)
  [Qes2] -> normalized_EML_power/2(Qes2)
  [Ils2] -> normalized_EML_power/3(Ils2)
  [Qls2] -> normalized_EML_power/4(Qls2)
  EML_power/1(Out) -> Mux/3
  normalized_EML_power/1(Out) -> Mux/4
  coherent_discriminator/1 -> Mux/2
  Mux/1 -> sdfa/1

== system tracker/code_carrier_tracking_loop1/carrier_loop_discriminator/loop_filter/digital_bilinear_z_transform_integrator ==
  x[n] : Inport
  AddSub : xbsIndex_r4/AddSub  mode=Addition  use_carryin=off  use_carryout=off  en=off  latency=0  precision=Full  arith_type=Unsigned  n_bits=16  bin_pt=14  quantization=Truncate  overflow=Wrap  use_behavioral_HDL=off  hw_selection=Fabric  pipelined=off  dbl_ovrd=off  block_type=addsub
  AddSub1 : xbsIndex_r4/AddSub  mode=Addition  use_carryin=off  use_carryout=off  en=off  latency=0  precision=Full  arith_type=Unsigned  n_bits=16  bin_pt=14  quantization=Truncate  overflow=Wrap  use_behavioral_HDL=off  hw_selection=Fabric  pipelined=off  dbl_ovrd=off  block_type=addsub
  CMult : xbsIndex_r4/CMult  const=1  gui_display_data_type=Fixed-point  const_n_bits=16  const_bin_pt=14  float_type=Single  exp_bits=8  fraction_bits=24  en=off  latency=1  precision=Full  arith_type="Signed  (2's comp)"  n_bits=16  bin_pt=14  quantization=Truncate  overflow=Wrap  use_behavioral_HDL=off  mem_type=Distributed RAM  pipeline=off  dbl_ovrd=off  block_type=cmult
  Register : xbsIndex_r4/Register  init=0  rst=off  en=off  dbl_ovrd=off  block_type=register
  Shift : xbsIndex_r4/Shift  shift_dir=Right  shift_bits=1  en=off  latency=0  precision=Full  arith_type="Signed  (2's comp)"  n_bits=16  bin_pt=14  quantization=Truncate  overflow=Wrap  dbl_ovrd=off  block_type=shift
  y[n] : Outport
  wires:
  AddSub/1 -> Register/1, AddSub1/1
  x[n]/1 -> CMult/1
  Register/1 -> AddSub/2, AddSub1/2
  AddSub1/1 -> Shift/1
  Shift/1 -> y[n]/1
  CMult/1 -> AddSub/1

== system tracker/code_carrier_tracking_loop1/carrier_loop_discriminator/loop_filter/digital_bilinear_z_transform_integrator1 ==
  x[n] : Inport
  AddSub : xbsIndex_r4/AddSub  mode=Addition  use_carryin=off  use_carryout=off  en=off  latency=0  precision=Full  arith_type=Unsigned  n_bits=16  bin_pt=14  quantization=Truncate  overflow=Wrap  use_behavioral_HDL=off  hw_selection=Fabric  pipelined=off  dbl_ovrd=off  block_type=addsub
  AddSub1 : xbsIndex_r4/AddSub  mode=Addition  use_carryin=off  use_carryout=off  en=off  latency=0  precision=Full  arith_type=Unsigned  n_bits=16  bin_pt=14  quantization=Truncate  overflow=Wrap  use_behavioral_HDL=off  hw_selection=Fabric  pipelined=off  dbl_ovrd=off  block_type=addsub
  CMult : xbsIndex_r4/CMult  const=1  gui_display_data_type=Fixed-point  const_n_bits=16  const_bin_pt=14  float_type=Single  exp_bits=8  fraction_bits=24  en=off  latency=1  precision=Full  arith_type="Signed  (2's comp)"  n_bits=16  bin_pt=14  quantization=Truncate  overflow=Wrap  use_behavioral_HDL=off  mem_type=Distributed RAM  pipeline=off  dbl_ovrd=off  block_type=cmult
  Register : xbsIndex_r4/Register  init=0  rst=off  en=off  dbl_ovrd=off  block_type=register
  Shift : xbsIndex_r4/Shift  shift_dir=Right  shift_bits=1  en=off  latency=0  precision=Full  arith_type="Signed  (2's comp)"  n_bits=16  bin_pt=14  quantization=Truncate  overflow=Wrap  dbl_ovrd=off  block_type=shift
  y[n] : Outport
  wires:
  CMult/1 -> AddSub/1
  Shift/1 -> y[n]/1
  AddSub1/1 -> Shift/1
  Register/1 -> AddSub1/2, AddSub/2
  x[n]/1 -> CMult/1
  AddSub/1 -> AddSub1/1, Register/1

== system tracker/code_carrier_tracking_loop1/carrier_loop_discriminator/loop_filter/digital_bilinear_z_transform_integrator2 ==
  x[n] : Inport
  AddSub : xbsIndex_r4/AddSub  mode=Addition  use_carryin=off  use_carryout=off  en=off  latency=0  precision=Full  arith_type=Unsigned  n_bits=16  bin_pt=14  quantization=Truncate  overflow=Wrap  use_behavioral_HDL=off  hw_selection=Fabric  pipelined=off  dbl_ovrd=off  block_type=addsub
  AddSub1 : xbsIndex_r4/AddSub  mode=Addition  use_carryin=off  use_carryout=off  en=off  latency=0  precision=Full  arith_type=Unsigned  n_bits=16  bin_pt=14  quantization=Truncate  overflow=Wrap  use_behavioral_HDL=off  hw_selection=Fabric  pipelined=off  dbl_ovrd=off  block_type=addsub
  CMult : xbsIndex_r4/CMult  const=1  gui_display_data_type=Fixed-point  const_n_bits=16  const_bin_pt=14  float_type=Single  exp_bits=8  fraction_bits=24  en=off  latency=1  precision=Full  arith_type="Signed  (2's comp)"  n_bits=16  bin_pt=14  quantization=Truncate  overflow=Wrap  use_behavioral_HDL=off  mem_type=Distributed RAM  pipeline=off  dbl_ovrd=off  block_type=cmult
  Register : xbsIndex_r4/Register  init=0  rst=off  en=off  dbl_ovrd=off  block_type=register
  Shift : xbsIndex_r4/Shift  shift_dir=Right  shift_bits=1  en=off  latency=0  precision=Full  arith_type="Signed  (2's comp)"  n_bits=16  bin_pt=14  quantization=Truncate  overflow=Wrap  dbl_ovrd=off  block_type=shift
  y[n] : Outport
  wires:
  CMult/1 -> AddSub/1
  Shift/1 -> y[n]/1
  AddSub1/1 -> Shift/1
  Register/1 -> AddSub1/2, AddSub/2
  x[n]/1 -> CMult/1
  AddSub/1 -> AddSub1/1, Register/1

== system tracker/code_carrier_tracking_loop1/carrier_loop_discriminator/pll_discriminators/costas_pll_QI ==
  I : Inport
  Q : Inport  Port=2
  Mult : xbsIndex_r4/Mult  precision=User Defined  arith_type="Signed  (2's comp)"  n_bits=costas_pll_QI_width  bin_pt=costas_pll_QI_point  quantization="Round  (unbiased: +/- Inf)"  overflow=Saturate  en=off  latency=3  use_behavioral_HDL=off  opt=Speed  use_embedded=on  optimum_pipeline=off  pipeline=on  dbl_ovrd=off  use_rpm=on  placement_style=Triangular  block_type=mult
  sin(2*phi) : Outport
  wires:
  Q/1 -> Mult/2
  I/1 -> Mult/1
  Mult/1 -> sin(2*phi)/1

== system tracker/code_carrier_tracking_loop1/carrier_loop_discriminator/pll_discriminators/costas_pll_arctan ==
  I : Inport
  Q : Inport  Port=2
  CORDIC ATAN : Subsystem  mask(Xilinx CORDIC ATAN){stages=costas_pll_arctan_nstage, pe_nbits=costas_pll_arctan_width, pe_binpt=costas_pll_arctan_point, pipeline_x=ones(1,costas_pll_arctan_nstage+1), prev_stages=8, pipeline=[1  1  1  1  1  1  1  1]}
      mask prompts: stages "Number of Processing Elements (integer value starting from 1)"; pe_nbits "X, Y Data Width"; pe_binpt "X, Y Binary Point Position"; pipeline_x "Latency for each Processing Element [1 0 0 1]"; prev_stages "Previous Number of Stages"; pipeline "Previous Pipeline Values"
      mask help: A parallel implementation, circular vectoring mode CORDIC processor for performing rectangular-to-polar conversion. The number of iteration stages (and resultant output accuracy) and the processor arithmetic precision are controlled by the mask customization.
      mask init:
      | [bg,fg] = xlcmap('XBlock',0);
      | iPos = get_param(gcb,'Position');
      | iWidth=iPos(3)-iPos(1); iHeight=iPos(4)-iPos(2);
      | iCx=iWidth/2;
      | iCy=iHeight/2;
      | [logoX, logoY] = xlogo(iPos);
      | sav_gcb=gcb;
      | stages = round(sum(abs(stages)));
      | if (stages == 0)
      | 	stages = prev_stages;
      | end
      | x = zeros(1,stages);
      | pipe_size = max(size(pipeline_x));
      | if pipe_size >= stages
      | 	x(1,1:stages) = pipeline_x(1,1:stages);
      | else
      | 	x(1,1:pipe_size) = pipeline_x(1,1:pipe_size);
      | end
      | 
      | if (stages ~=prev_stages)
      | 	pipeline=x;
      | 	cordic_pe = find_system(gcb, 'lookUnderMasks', 'all', 'FollowLinks','on','masktype', 'CORDIC parallel PE');
      |     
      |   a=find_system(cordic_pe{1}, 'lookUnderMasks', 'all', 'FollowLinks','on','masktype', 'CORDIC iteration PE');
      |   for i= 2:length(a)
      |     for j=1:3
      | 	  delete_line(cordic_pe{1}, ['CORDIC PE' int2str(i-1) '/' int2str(j)], ['CORDIC PE' int2str(i) '/' int2str(j)]);
      |     end
      |   end
      |     if length(a)>0,
      |       delete_line(cordic_pe{1}, 'x/1', 'CORDIC PE1/1');
      |       delete_line(cordic_pe{1}, 'y/1', 'CORDIC PE1/2');
      |       delete_line(cordic_pe{1}, 'z/1', 'CORDIC PE1/3');
      |       delete_line(cordic_pe{1}, ['CORDIC PE' int2str(length(a)) '/1'],'X/1');
      |       delete_line(cordic_pe{1}, ['CORDIC PE' int2str(length(a)) '/2'],'Terminator/1');
      |       delete_line(cordic_pe{1}, ['CORDIC PE' int2str(length(a)) '/3'],'Z/1');
      |     elseif length(a)==0
      |       temp_port=get_param([cordic_pe{1} '/x'],'porthandles');
      |       temp_line=get_param(temp_port.Outport,'line');
      |       if temp_line>=0  delete_line(temp_line); end
      |       temp_port=get_param([cordic_pe{1} '/y'],'porthandles');
      |       temp_line=get_param(temp_port.Outport,'line');
      |       if temp_line>=0  delete_line(temp_line); end
      |       temp_port=get_param([cordic_pe{1} '/z'],'porthandles');
      |       temp_line=get_param(temp_port.Outport,'line');
      |       if temp_line>=0  delete_line(temp_line); end
      |     end
      | 
      |     for i=2:length(a)
      |       delete_block(a{i});
      |     end
      |     for i=2:stages,
      |         add_block([cordic_pe{1} '/CORDIC PE1'], [cordic_pe{1} '/CORDIC PE' int2str(i)], 'ii', int2str(i-1),'pe_nbits', 'pe_nbits','pe_binpt', 'pe_binpt','pipeline',['pipeline(1,' int2str(i) ')'],'position',[150+(i-1)*125, 70, 205+(i-1)*125, 130]);
      |     end
      | 
      |     for i= 2:stages,
      |       for j=1:3
      | 		add_line(cordic_pe{1}, ['CORDIC PE' int2str(i-1) '/' int2str(j)], ['CORDIC PE' int2str(i) '/' int2str(j)], 'autorouting', 'on');
      |       end
      |     end
      | 
      |     if stages==0
      |       add_line(cordic_pe{1}, 'x/1', 'X/1', 'autorouting', 'on');
      |       add_line(cordic_pe{1}, 'y/1', 'Terminator/1', 'autorouting', 'on');
      |       add_line(cordic_pe{1}, 'z/1', 'Z/1', 'autorouting', 'on');
      |     elseif stages>0
      |       add_line(cordic_pe{1}, 'x/1', 'CORDIC PE1/1', 'autorouting', 'on');
      |       add_line(cordic_pe{1}, 'y/1', 'CORDIC PE1/2', 'autorouting', 'on');
      |       add_line(cordic_pe{1}, 'z/1', 'CORDIC PE1/3', 'autorouting', 'on');
      | 
      |       set_param([cordic_pe{1} '/' 'X'], 'Position', [150+stages*125, 72, 180+stages*125, 86]);
      |       set_param([cordic_pe{1} '/' 'Terminator'], 'Position', [210+stages*125, 92, 225+stages*125, 108]);
      |       set_param([cordic_pe{1} '/' 'Z'], 'Position', [240+stages*125, 113, 270+stages*125, 127]);
      | 
      |       add_line(cordic_pe{1}, ['CORDIC PE' int2str(stages) '/1'], 'X/1', 'autorouting', 'on');
      |       add_line(cordic_pe{1}, ['CORDIC PE' int2str(stages) '/2'], 'Terminator/1', 'autorouting', 'on');
      |       add_line(cordic_pe{1}, ['CORDIC PE' int2str(stages) '/3'],'Z/1', 'autorouting', 'on');
      | 
      |       % force a "compile" of the constituent constant blocks to
      |       % workaround a data propagation problem
      |       find_system(cordic_pe{1}, 'lookUnderMasks', 'all', 'FollowLinks', 'on', 'MaskType','Xilinx Constant Block');
      |   end
      | 	set_param(sav_gcb, 'prev_stages', int2str(stages));
      | 	set_param(sav_gcb, 'pipeline', [ '[' int2str(x) ']']);
      | else
      | 	if (sum(pipeline~=x))
      | 		set_param(gcb, 'pipeline', [ '[' int2str(x) ']']);
      | 	end
      | end
      | str = sprintf('-%d',sum(x) + 3);
      settings: CopyFcn=set_param(gcb, 'MaskSelfModifiable', 'on', 'LinkStatus', 'none');
      mask Help: eval('');xlDoc('-book','sysgen','-topic','CORDIC_ATAN');
      mask Display:
      | patch([0 iWidth iWidth 0],[0 0 iHeight iHeight] , bg);
      | patch(logoX,logoY , fg);
      | text(iCx-6,iCy,'z');
      | text(iCx,iCy+4,str);
      | port_label('input',1,'x');
      | port_label('input',2,'y');
      | port_label('output',1,'mag');
      | port_label('output',2,'atan');
      | plot([0 0 iWidth iWidth 0], [0 iHeight iHeight 0 0]);
  phi : Outport
  wires:
  I/1 -> CORDIC ATAN/1(x)
  CORDIC ATAN/2(Z) -> phi/1
  Q/1 -> CORDIC ATAN/2(y)

== system tracker/code_carrier_tracking_loop1/carrier_loop_discriminator/pll_discriminators/costas_pll_sign ==
  I : Inport
  Q : Inport  Port=2
  Mux : xbsIndex_r4/Mux  inputs=2  en=off  latency=1  precision=Full  arith_type=Unsigned  n_bits=16  bin_pt=14  quantization=Truncate  overflow=Wrap  dbl_ovrd=off  block_type=mux
  Negate : xbsIndex_r4/Negate  precision=User Defined  arith_type="Signed  (2's comp)"  n_bits=costas_pll_sign_width  bin_pt=costas_pll_sign_point  quantization="Round  (unbiased: +/- Inf)"  overflow=Saturate  en=off  latency=1  dbl_ovrd=off  block_type=negate
  sign : xbsIndex_r4/Slice  nbits=1  boolean_output=on  mode=Upper Bit Location + Width  bit1=0  base1=MSB of Input  bit0=0  base0=LSB of Input  dbl_ovrd=off  block_type=slice
  sin(phi) : Outport
  wires:
  sign/1 -> Mux/1
  I/1 -> sign/1
  Mux/1 -> sin(phi)/1
  Negate/1 -> Mux/3
  Q/1 -> Mux/2, Negate/1

== system tracker/code_carrier_tracking_loop1/code_loop_discriminator/DLL_Discriminators/EML_power ==
  Ies2 : Inport
  Qes2 : Inport  Port=2
  Ils2 : Inport  Port=3
  Qls2 : Inport  Port=4
  AddSub : xbsIndex_r4/AddSub  mode=Subtraction  use_carryin=off  use_carryout=off  en=off  latency=1  precision=User Defined  arith_type="Signed  (2's comp)"  n_bits=EML_power_sub_width  bin_pt=EML_power_sub_point  quantization="Round  (unbiased: +/- Inf)"  overflow=Saturate  use_behavioral_HDL=off  hw_selection=Fabric  pipelined=off  dbl_ovrd=off  block_type=addsub
  AddSub1 : xbsIndex_r4/AddSub  mode=Addition  use_carryin=off  use_carryout=off  en=off  latency=1  precision=User Defined  arith_type="Signed  (2's comp)"  n_bits=EML_power_add_width  bin_pt=EML_power_add_point  quantization="Round  (unbiased: +/- Inf)"  overflow=Saturate  use_behavioral_HDL=off  hw_selection=Fabric  pipelined=off  dbl_ovrd=off  block_type=addsub
  AddSub2 : xbsIndex_r4/AddSub  mode=Addition  use_carryin=off  use_carryout=off  en=off  latency=1  precision=User Defined  arith_type="Signed  (2's comp)"  n_bits=EML_power_add_width  bin_pt=EML_power_add_point  quantization="Round  (unbiased: +/- Inf)"  overflow=Saturate  use_behavioral_HDL=off  hw_selection=Fabric  pipelined=off  dbl_ovrd=off  block_type=addsub
  Out : Outport
  wires:
  Qes2/1 -> AddSub1/2
  Ies2/1 -> AddSub1/1
  Qls2/1 -> AddSub2/2
  Ils2/1 -> AddSub2/1
  AddSub1/1 -> AddSub/1
  AddSub2/1 -> AddSub/2
  AddSub/1 -> Out/1
